simulink model "exp2M_CSVPosRefCtrl"  (R2020a)
settings: Solver=FixedStepAuto  StartTime=0.0  StopTime=10  RelTol=1e-3
InitFcn:
  | %Motor1 = Epos4(1,0);
  | %Motor2 = Epos4(2,0);
  | load expsetup sm_posn
model workspace (MAT data in the model file):
  Ki1 = 3.68920166721
  Ki2 = 3.68940567793
  Kp1 = 0.00368920166721
  Kp2 = 0.00368940567793
undefined symbols (not defined in the file or in its folder): x607325_PPR
libraries: simulink x4
CloseFcn:
  | %delete(Motor1);
  | %delete(Motor2);
settings Model: DataDictionary=MotorInfo.sldd  SimulationMode=accelerator  Creator=khoi  LastModifiedBy=khoi
settings DataIOCC: InspectSignalLogs=on
settings OptimizationCC: EfficientMapNaN2IntZero=off
settings HardwareCC: TargetBitPerPointer=64  TargetBitPerSizeT=64  TargetBitPerPtrDiffT=64  TargetLongLongMode=on  TargetIntDivRoundTo=Zero  TargetEndianess=LittleEndian  TargetWordSize=64  TargetHWDeviceType=MATLAB Host  ProdEqTarget=off
settings CodeAppCC: MaxIdLength=128
settings GRTTargetCC: CombineOutputUpdateFcns=off  GRTInterface=on

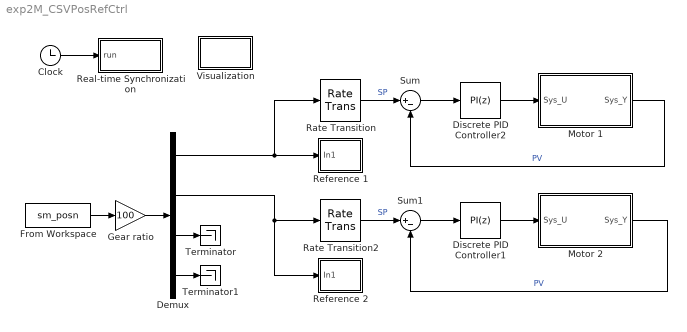
== system exp2M_CSVPosRefCtrl ==
  Clock : Clock
  Demux : Demux
  Discrete PID Controller1 : simulink/Continuous/PID Controller  Controller=PI  Form=Parallel  TimeDomain=Discrete-time  UseExternalTs=off  SampleTime=2e-3  IntegratorMethod=Forward Euler  FilterMethod=Forward Euler  ControllerParametersSource=internal  P=Kp2  I=Ki2  D=0  UseFilter=on  N=100  TunerSelectOption=Transfer Function Based (PID Tuner App)  InitialConditionSource=internal  InitialConditionForIntegrator=0  InitialConditionForFilter=0  DifferentiatorICPrevScaledInput=0  ExternalReset=none  TrackingMode=off  Kt=1  LimitOutput=off  UpperSaturationLimit=2000  LowerSaturationLimit=-2000  LinearizeAsGain=off  AntiWindupMode=clamping  Kb=1  POutMin=[]  POutMax=[]  IOutMin=[]  IOutMax=[]  DOutMin=[]  DOutMax=[]  NOutMin=[]  NOutMax=[]  SumOutMin=[]  SumOutMax=[]  SaturationOutMin=[]  SaturationOutMax=[]  PParamMin=[]  PParamMax=[]  IParamMin=[]  IParamMax=[]  DParamMin=[]  DParamMax=[]  NParamMin=[]  NParamMax=[]  KbParamMin=[]  KbParamMax=[]  KtParamMin=[]  KtParamMax=[]  KbOutMin=[]  KbOutMax=[]  KtOutMin=[]  KtOutMax=[]  IntegratorOutMin=[]  IntegratorOutMax=[]  FilterOutMin=[]  FilterOutMax=[]  SumI1OutMin=[]  SumI1OutMax=[]  SumI2OutMin=[]  SumI2OutMax=[]  SumI3OutMin=[]  SumI3OutMax=[]  SumI4OutMin=[]  SumI4OutMax=[]  SumDOutMin=[]  SumDOutMax=[]  DifferentiatorOutMin=[]  DifferentiatorOutMax=[]  FilterDiffOutCoefMin=[]  FilterDiffOutCoefMax=[]  ReciprocalOutMin=[]  ReciprocalOutMax=[]  SumDenOutMin=[]  SumDenOutMax=[]  SumNumOutMin=[]  SumNumOutMax=[]  DivideOutMin=[]  DivideOutMax=[]  UdiffTsProdOutMin=[]  UdiffTsProdOutMax=[]  NTsProdOutMin=[]  NTsProdOutMax=[]  UintegralTsProdOutMin=[]  UintegralTsProdOutMax=[]  UngainTsProdOutMin=[]  UngainTsProdOutMax=[]  IntegratorContinuousStateAttributes=''  IntegratorStateMustResolveToSignalObject=off  IntegratorRTWStateStorageClass=Auto  FilterContinuousStateAttributes=''  FilterStateMustResolveToSignalObject=off  FilterRTWStateStorageClass=Auto  ParallelPVariant=InternalParameters  IdealPVariant=Disabled  IVariant=InternalParameters  DVariant=Disabled  IntegratorVariant=Discrete  SatVariant=Disabled  AWVariant=Passthrough  PCopyVariant=Disabled  TRVariant=Disabled  FdbkBlocksVariant=Forward  IdealPFdbkVariant=Disabled  SatFdbkVariant=Disabled  DerivativeFilterVariant=Disabled  NVariant=Disabled  NCopyVariant=Disabled_SignalSpec  FilterICVariant=Disabled  IntegratorICVariant=InternalICs  ExternalResetVariant=Disabled  TRSumVariant=Passthrough  SumFdbkVariant=Disabled  SumVariant=Sum_PI  TsampFilterVariant=InternalTs  TsampNgainVariant=Passthrough  TsampIntegralVariant=Passthrough
  Discrete PID Controller2 : simulink/Continuous/PID Controller  Controller=PI  Form=Parallel  TimeDomain=Discrete-time  UseExternalTs=off  SampleTime=2e-3  IntegratorMethod=Forward Euler  FilterMethod=Forward Euler  ControllerParametersSource=internal  P=Kp1  I=Ki1  D=0  UseFilter=on  N=100  TunerSelectOption=Transfer Function Based (PID Tuner App)  InitialConditionSource=internal  InitialConditionForIntegrator=0  InitialConditionForFilter=0  DifferentiatorICPrevScaledInput=0  ExternalReset=none  TrackingMode=off  Kt=1  LimitOutput=off  UpperSaturationLimit=2000  LowerSaturationLimit=-2000  LinearizeAsGain=off  AntiWindupMode=clamping  Kb=1  POutMin=[]  POutMax=[]  IOutMin=[]  IOutMax=[]  DOutMin=[]  DOutMax=[]  NOutMin=[]  NOutMax=[]  SumOutMin=[]  SumOutMax=[]  SaturationOutMin=[]  SaturationOutMax=[]  PParamMin=[]  PParamMax=[]  IParamMin=[]  IParamMax=[]  DParamMin=[]  DParamMax=[]  NParamMin=[]  NParamMax=[]  KbParamMin=[]  KbParamMax=[]  KtParamMin=[]  KtParamMax=[]  KbOutMin=[]  KbOutMax=[]  KtOutMin=[]  KtOutMax=[]  IntegratorOutMin=[]  IntegratorOutMax=[]  FilterOutMin=[]  FilterOutMax=[]  SumI1OutMin=[]  SumI1OutMax=[]  SumI2OutMin=[]  SumI2OutMax=[]  SumI3OutMin=[]  SumI3OutMax=[]  SumI4OutMin=[]  SumI4OutMax=[]  SumDOutMin=[]  SumDOutMax=[]  DifferentiatorOutMin=[]  DifferentiatorOutMax=[]  FilterDiffOutCoefMin=[]  FilterDiffOutCoefMax=[]  ReciprocalOutMin=[]  ReciprocalOutMax=[]  SumDenOutMin=[]  SumDenOutMax=[]  SumNumOutMin=[]  SumNumOutMax=[]  DivideOutMin=[]  DivideOutMax=[]  UdiffTsProdOutMin=[]  UdiffTsProdOutMax=[]  NTsProdOutMin=[]  NTsProdOutMax=[]  UintegralTsProdOutMin=[]  UintegralTsProdOutMax=[]  UngainTsProdOutMin=[]  UngainTsProdOutMax=[]  IntegratorContinuousStateAttributes=''  IntegratorStateMustResolveToSignalObject=off  IntegratorRTWStateStorageClass=Auto  FilterContinuousStateAttributes=''  FilterStateMustResolveToSignalObject=off  FilterRTWStateStorageClass=Auto  ParallelPVariant=InternalParameters  IdealPVariant=Disabled  IVariant=InternalParameters  DVariant=Disabled  IntegratorVariant=Discrete  SatVariant=Disabled  AWVariant=Passthrough  PCopyVariant=Disabled  TRVariant=Disabled  FdbkBlocksVariant=Forward  IdealPFdbkVariant=Disabled  SatFdbkVariant=Disabled  DerivativeFilterVariant=Disabled  NVariant=Disabled  NCopyVariant=Disabled_SignalSpec  FilterICVariant=Disabled  IntegratorICVariant=InternalICs  ExternalResetVariant=Disabled  TRSumVariant=Passthrough  SumFdbkVariant=Disabled  SumVariant=Sum_PI  TsampFilterVariant=InternalTs  TsampNgainVariant=Passthrough  TsampIntegralVariant=Passthrough
  From Workspace : FromWorkspace  VariableName=sm_posn
  Gear ratio : Gain  Gain=100
  Motor 1 : Subsystem
  Motor 2 : Subsystem
  Rate Transition : RateTransition  OutPortSampleTime=0.02
  Rate Transition2 : RateTransition  OutPortSampleTime=0.02
  Real-time Synchronization : Subsystem
  Reference 1 : Subsystem
  Reference 2 : Subsystem
  Sum : Sum  Inputs=|+-
  Sum1 : Sum  Inputs=|+-
  Terminator : Terminator
  Terminator1 : Terminator
  Visualization : Subsystem
  wires:
  Clock/1 -> Real-time Synchronization/1(run)
  Demux/1 -> Rate Transition/1, Reference 1/1(In1)
  Sum/1 -> Discrete PID Controller2/1
  Sum1/1 -> Discrete PID Controller1/1
  From Workspace/1 -> Gear ratio/1
  Demux/3 -> Terminator/1
  Demux/4 -> Terminator1/1
  Gear ratio/1 -> Demux/1
  Rate Transition/1 -> Sum/1  "SP"
  Discrete PID Controller2/1 -> Motor 1/1(Sys_U)
  Motor 1/1(Sys_Y) -> Sum/2  "PV"
  Discrete PID Controller1/1 -> Motor 2/1(Sys_U)
  Motor 2/1(Sys_Y) -> Sum1/2  "PV"
  Rate Transition2/1 -> Sum1/1  "SP"
  Demux/2 -> Reference 2/1(In1), Rate Transition2/1

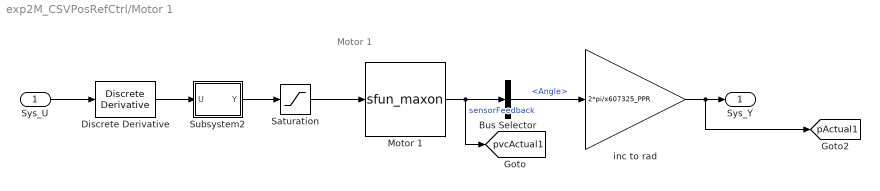
== system exp2M_CSVPosRefCtrl/Motor 1 ==
  note: Motor 1
  Sys_U : Inport
  Bus Selector : BusSelector  OutputSignals=Angle
  Discrete Derivative : simulink/Discrete/Discrete Derivative  gainval=1.0  ICPrevScaledInput=0.0  OutMin=[]  OutMax=[]  OutDataType=fixdt(1, 16)  OutScaling=2^-10  DoSatur=off
  Motor 1 : S-Function  FunctionName=sfun_maxon  Parameters=NodeID, DeltaT, OpMode  SFunctionDeploymentMode=off  EnableBusSupport=off  mask{NodeID=1, DeltaT=0.02, OpMode=Cyclic synchronous velocity mode, P_cur=0, I_cur=0, P_pos=0, I_pos=0, D_pos=0, v_posGainFF=0, a_posGainFF=0, P_vel=0, I_vel=0, v_velGainFF=0, a_velGainFF=0, f_velCutoff=0}
      mask prompts: NodeID "Node ID"; DeltaT "Sample time (s)"; OpMode "Operation mode"; P_cur "P gain"; I_cur "I gain"; P_pos "P gain"; I_pos "I gain"; D_pos "D gain"; v_posGainFF "FF velocity gain"; a_posGainFF "FF acceleration gain"; P_vel "P gain"; I_vel "I gain"; v_velGainFF "Feed-forward velocity gain"; a_velGainFF "Feed-forward acceleration gain"; f_velCutoff "Filter cut-off frequency"
      mask TypeOptions OpMode: Cyclic synchronous current (torque) mode | Cyclic synchronous velocity mode | Cyclic synchronous position mode | Profile velocity mode | Profile position mode
      mask DialogControl DescGroupVar Prompt: Motor Parameters
      mask DialogControl DescTextVar Prompt: The block outputs MotorInfo bus signal, which consists of the following variables: angle (increment), speed (rpm), current (mA)
      mask DialogControl Container6 Prompt: Motor
      mask DialogControl Container14 Prompt: Controller Parameters
      mask DialogControl DescTextVar_copy Prompt: This tab is experimental and does not implemented yet. Changing these parameters will not affect the motor performance.
      mask DialogControl Container15 Prompt: Current controller parameter set
      mask DialogControl Container15_copy Prompt: Position controller parameter set
      mask DialogControl Container15_copy_copy Prompt: Velocity controller parameter set
      mask Display:
      | disp('Maxon motor\nHIL');
      | % port_label('input', 1, 'inputSignal');
      | % port_label('output', 1, 'SENSR');
  Saturation : Saturate  UpperLimit=2000  LowerLimit=-2000
  Subsystem2 : Subsystem
      mask Display: disp('To rpm')
  inc to rad : Gain  Gain=2*pi/x607325_PPR
  Sys_Y : Outport
  tag scope: pActual1=global, pvcActual1=global
  wires:
  Subsystem2/1(Y) -> Saturation/1
  Discrete Derivative/1 -> Subsystem2/1(U)
  Saturation/1 -> Motor 1/1
  Motor 1/1 -> [pvcActual1], Bus Selector/1  "sensorFeedback"
  Sys_U/1 -> Discrete Derivative/1
  Bus Selector/1 -> inc to rad/1  "<Angle>"
  inc to rad/1 -> Sys_Y/1, [pActual1]

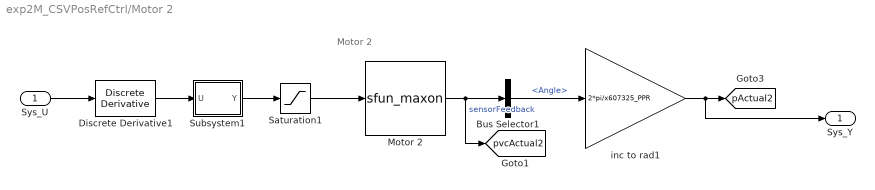
== system exp2M_CSVPosRefCtrl/Motor 2 ==
  note: Motor 2
  Sys_U : Inport
  Bus Selector1 : BusSelector  OutputSignals=Angle
  Discrete Derivative1 : simulink/Discrete/Discrete Derivative  gainval=1.0  ICPrevScaledInput=0.0  OutMin=[]  OutMax=[]  OutDataType=fixdt(1, 16)  OutScaling=2^-10  DoSatur=off
  Motor 2 : S-Function  FunctionName=sfun_maxon  Parameters=NodeID, DeltaT, OpMode  SFunctionDeploymentMode=off  EnableBusSupport=off  mask{NodeID=2, DeltaT=0.02, OpMode=Profile velocity mode, P_cur=0, I_cur=0, P_pos=0, I_pos=0, D_pos=0, v_posGainFF=0, a_posGainFF=0, P_vel=0, I_vel=0, v_velGainFF=0, a_velGainFF=0, f_velCutoff=0}
      mask prompts: NodeID "Node ID"; DeltaT "Sample time (s)"; OpMode "Operation mode"; P_cur "P gain"; I_cur "I gain"; P_pos "P gain"; I_pos "I gain"; D_pos "D gain"; v_posGainFF "FF velocity gain"; a_posGainFF "FF acceleration gain"; P_vel "P gain"; I_vel "I gain"; v_velGainFF "Feed-forward velocity gain"; a_velGainFF "Feed-forward acceleration gain"; f_velCutoff "Filter cut-off frequency"
      mask TypeOptions OpMode: Cyclic synchronous current (torque) mode | Cyclic synchronous velocity mode | Cyclic synchronous position mode | Profile velocity mode | Profile position mode
      mask DialogControl DescGroupVar Prompt: Motor Parameters
      mask DialogControl DescTextVar Prompt: The block outputs MotorInfo bus signal, which consists of the following variables: angle (increment), speed (rpm), current (mA)
      mask DialogControl Container6 Prompt: Motor
      mask DialogControl Container14 Prompt: Controller Parameters
      mask DialogControl DescTextVar_copy Prompt: This tab is experimental and does not implemented yet. Changing these parameters will not affect the motor performance.
      mask DialogControl Container15 Prompt: Current controller parameter set
      mask DialogControl Container15_copy Prompt: Position controller parameter set
      mask DialogControl Container15_copy_copy Prompt: Velocity controller parameter set
      mask Display:
      | disp('Maxon motor\nHIL');
      | % port_label('input', 1, 'inputSignal');
      | % port_label('output', 1, 'SENSR');
  Saturation1 : Saturate  UpperLimit=2000  LowerLimit=-2000
  Subsystem1 : Subsystem
      mask Display: disp('To rpm')
  inc to rad1 : Gain  Gain=2*pi/x607325_PPR
  Sys_Y : Outport
  tag scope: pActual2=global, pvcActual2=global
  wires:
  Saturation1/1 -> Motor 2/1
  Subsystem1/1(Y) -> Saturation1/1
  Discrete Derivative1/1 -> Subsystem1/1(U)
  Sys_U/1 -> Discrete Derivative1/1
  Bus Selector1/1 -> inc to rad1/1  "<Angle>"
  inc to rad1/1 -> Sys_Y/1, [pActual2]
  Motor 2/1 -> [pvcActual2], Bus Selector1/1  "sensorFeedback"

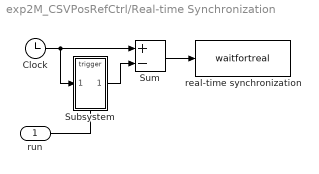
== system exp2M_CSVPosRefCtrl/Real-time Synchronization ==
  run : Inport
  Clock : Clock
  Subsystem : Subsystem  TreatAsAtomicUnit=on
  Sum : Sum  Inputs=+-  InputSameDT=on  SaturateOnIntegerOverflow=on  OutDataTypeStr=Inherit: Same as first input
  real-time synchronization : MATLABFcn  MATLABFcn=waitfortreal  OutputDimensions=0
  wires:
  Clock/1 -> Subsystem/1(In), Sum/1
  Subsystem/1(Out) -> Sum/2
  Sum/1 -> real-time synchronization/1
  run/1 -> Subsystem/Trigger

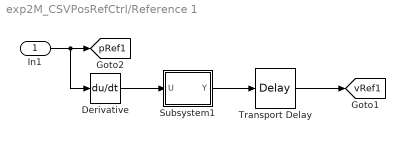
== system exp2M_CSVPosRefCtrl/Reference 1 ==
  In1 : Inport
  Derivative : Derivative
  Subsystem1 : Subsystem
      mask Display: disp('To rpm')
  Transport Delay : TransportDelay  DelayTime=0.1
  tag scope: pRef1=global, vRef1=global
  wires:
  Subsystem1/1(Y) -> Transport Delay/1
  Derivative/1 -> Subsystem1/1(U)
  In1/1 -> Derivative/1, [pRef1]
  Transport Delay/1 -> [vRef1]

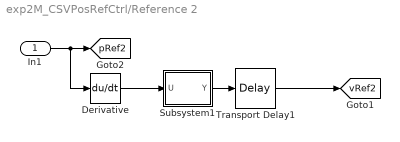
== system exp2M_CSVPosRefCtrl/Reference 2 ==
  In1 : Inport
  Derivative : Derivative
  Subsystem1 : Subsystem
      mask Display: disp('To rpm')
  Transport Delay1 : TransportDelay  DelayTime=0.1
  tag scope: pRef2=global, vRef2=global
  wires:
  Subsystem1/1(Y) -> Transport Delay1/1
  In1/1 -> [pRef2], Derivative/1
  Derivative/1 -> Subsystem1/1(U)
  Transport Delay1/1 -> [vRef2]

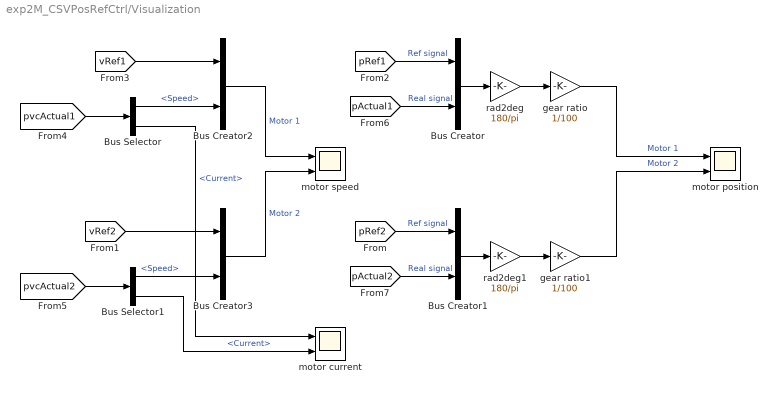
== system exp2M_CSVPosRefCtrl/Visualization ==
  Bus Selector : BusSelector  OutputSignals=Speed,Current
  Bus Selector1 : BusSelector  OutputSignals=Speed,Current
  Bus Creator{,1..3} (4 alike) : BusCreator  Inputs=2
  gear ratio : Gain  Gain=1/100
  gear ratio1 : Gain  Gain=1/100
  motor current : Scope  NumInputPorts=2
  motor position : Scope  NumInputPorts=2
  motor speed : Scope  NumInputPorts=2
  rad2deg : Gain  Gain=180/pi
  rad2deg1 : Gain  Gain=180/pi
  wires:
  [pvcActual2] -> Bus Selector1/1
  [pvcActual1] -> Bus Selector/1
  Bus Selector/2 -> motor current/1  "<Current>"
  Bus Selector1/2 -> motor current/2  "<Current>"
  [pRef1] -> Bus Creator/1  "Ref signal"
  [pActual1] -> Bus Creator/2  "Real signal"
  Bus Creator/1 -> rad2deg/1
  gear ratio/1 -> motor position/1  "Motor 1"
  [pRef2] -> Bus Creator1/1  "Ref signal"
  [pActual2] -> Bus Creator1/2  "Real signal"
  Bus Creator1/1 -> rad2deg1/1
  gear ratio1/1 -> motor position/2  "Motor 2"
  rad2deg/1 -> gear ratio/1
  rad2deg1/1 -> gear ratio1/1
  [vRef1] -> Bus Creator2/1
  Bus Selector/1 -> Bus Creator2/2  "<Speed>"
  Bus Creator2/1 -> motor speed/1  "Motor 1"
  [vRef2] -> Bus Creator3/1
  Bus Selector1/1 -> Bus Creator3/2  "<Speed>"
  Bus Creator3/1 -> motor speed/2  "Motor 2"

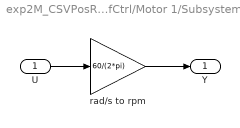
== system exp2M_CSVPosRefCtrl/Motor 1/Subsystem2 ==
  U : Inport
  rad/s to rpm : Gain  Gain=60/(2*pi)
  Y : Outport
  wires:
  U/1 -> rad/s to rpm/1
  rad/s to rpm/1 -> Y/1

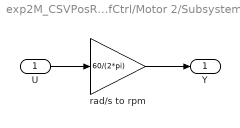
== system exp2M_CSVPosRefCtrl/Motor 2/Subsystem1 ==
  U : Inport
  rad/s to rpm : Gain  Gain=60/(2*pi)
  Y : Outport
  wires:
  rad/s to rpm/1 -> Y/1
  U/1 -> rad/s to rpm/1

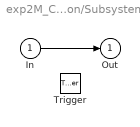
== system exp2M_CSVPosRefCtrl/Real-time Synchronization/Subsystem ==
  In : Inport
  Trigger : TriggerPort  VariantControl=(inherit)
  Out : Outport  InitialOutput=0
  wires:
  In/1 -> Out/1

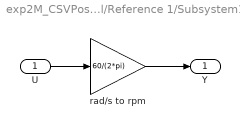
== system exp2M_CSVPosRefCtrl/Reference 1/Subsystem1 ==
  U : Inport
  rad/s to rpm : Gain  Gain=60/(2*pi)
  Y : Outport
  wires:
  rad/s to rpm/1 -> Y/1
  U/1 -> rad/s to rpm/1

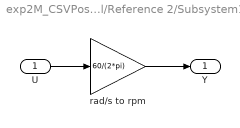
== system exp2M_CSVPosRefCtrl/Reference 2/Subsystem1 ==
  U : Inport
  rad/s to rpm : Gain  Gain=60/(2*pi)
  Y : Outport
  wires:
  rad/s to rpm/1 -> Y/1
  U/1 -> rad/s to rpm/1
